simulink model "Three_Phase_Rectifier"  (R2019b)
settings: Solver=ode45  StartTime=0.0  StopTime=2  RelTol=1e-3  EnableMultiTasking=on
libraries: powerlib x21, powerlib_extras x4, eeTransforms x1, simulink x1
settings Model: Creator=Administrator  LastModifiedBy=de
settings DataIOCC: LimitDataPoints=on  SaveFormat=Array  SignalLoggingSaveFormat=ModelDataLogs  ReturnWorkspaceOutputs=off
settings OptimizationCC: ExpressionDepthLimit=2147483647  LifeSpan=inf
settings DebuggingCC: UnderspecifiedInitializationDetection=Classic  MergeDetectMultiDrivingBlocksExec=none  SolverPrmCheckMsg=warning  FcnCallInpInsideContextMsg=warning  StateNameClashWarn=warning  SFUnexpectedBacktrackingDiag=warning  SFNoUnconditionalDefaultTransitionDiag=warning  SFExecutionAtInitializationDiag=none  ArithmeticOperatorsInVariantConditions=warning
settings HardwareCC: ProdBitPerPointer=32  ProdBitPerSizeT=32  ProdBitPerPtrDiffT=32  ProdLargestAtomicFloat=None  ProdIntDivRoundTo=Undefined  ProdEndianess=Unspecified  ProdWordSize=32  ProdHWDeviceType=32-bit Generic
settings ModelReferenceCC: PropagateSignalLabelsOutOfModel=off
settings SFSimCC: SimUseLocalCustomCode=off  CustomCodeUndefinedFunction=UseInterfaceOnly
settings RTWCC: RTWUseLocalCustomCode=off
settings CodeAppCC: StateflowObjectComments=on
settings GRTTargetCC: TargetLangStandard=C89/C90 (ANSI)  GeneratePreprocessorConditionals=Disable all  CombineOutputUpdateFcns=off  GRTInterface=on
settings ConfigComp: CovMetricSettings=dw  CovHtmlReporting=on  CovSaveCumulativeToWorkspaceVar=on  CovSaveSingleToWorkspaceVar=on  CovExternalEMLEnable=off
settings SimscapeCC: SimscapeNormalizeSystem=off

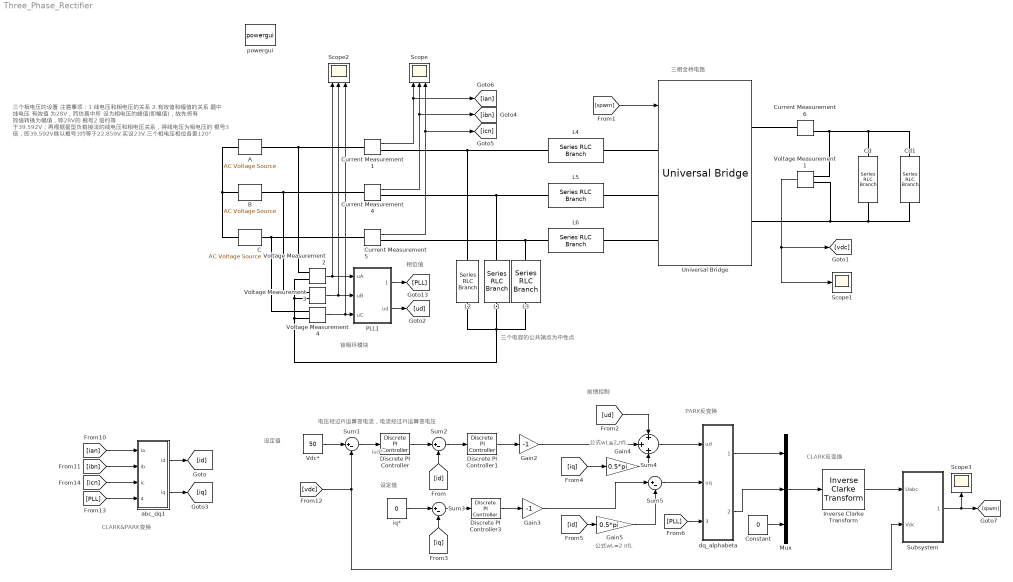
== system Three_Phase_Rectifier ==
  note: 前馈控制
  note: 电压经过PI运算变电流，电流经过PI运算变电压
  note: 公式wL=2 πfL
  note: 相位值
  note: 设定值
  note: CLARK&PARK变换
  note: PARK反变换
  note: 三个电容的公共端点为中性点
  note: isd*
  note: 三个相电压的设置
      | 注意事项：1.线电压和相电压的关系
      | 2.有效值和幅值的关系
      | 题中 线电压 有效值 为28V，而仿真中所
      | 设为相电压的峰值(即幅值)，故先将有
      | 效值转换为幅值，即28V的 根号2 倍约等
      | 于39.592V；再根据星型负载接法的线电压和相电压关系，得线电压为相电压的 根号3 倍，即39.592V除以根号3约等于22.859V,实设23V.三个相电压相位各差120°
  note: 锁相环模块
  note: 三相全桥电路
  note: CLARK反变换
  note: 设定值
  note: 公式wL=2 πfL
  A : powerlib/Electrical Sources/AC Voltage Source  Amplitude=23  Phase=-120  Frequency=50  SampleTime=0  Measurements=None  BusType=swing  Pref=10e3  Qref=0  Qmin=-inf  Qmax=+inf
      settings: SourceProductName=Simscape Electrical
  B : powerlib/Electrical Sources/AC Voltage Source  Amplitude=23  Phase=120  Frequency=50  SampleTime=0  Measurements=None  BusType=swing  Pref=10e3  Qref=0  Qmin=-inf  Qmax=+inf
      settings: SourceProductName=Simscape Electrical
  C : powerlib/Electrical Sources/AC Voltage Source  Amplitude=23  Phase=0  Frequency=50  SampleTime=0  Measurements=None  BusType=swing  Pref=10e3  Qref=0  Qmin=-inf  Qmax=+inf
      settings: SourceProductName=Simscape Electrical
  Cd : powerlib/Elements/Series RLC Branch  LConnTagsString=__new0  RConnTagsString=__new0  BranchType=C  Resistance=100  Inductance=1e-3  SetiL0=off  InitialCurrent=0  Capacitance=1e-3  Setx0=on  InitialVoltage=0  Measurements=None
      settings: SourceProductName=Simscape Electrical
  Cd1 : powerlib/Elements/Series RLC Branch  LConnTagsString=__new0  RConnTagsString=__new0  BranchType=R  Resistance=50  Inductance=1e-3  SetiL0=off  InitialCurrent=0  Capacitance=2e-3  Setx0=on  InitialVoltage=540  Measurements=None
      settings: SourceProductName=Simscape Electrical
  Constant : Constant  Value=0
  Current Measurement{1,4..6} (4 alike) : powerlib/Measurements/Current Measurement  PhasorSimulation=off  OutputType=Complex  PSBequivalent=0
      settings: SourceProductName=Simscape Electrical
  Discrete PI Controller : powerlib_extras/Discrete  Control Blocks/Discrete PI Controller  Kp=0.5  Ki=12  Par_Limits=[30 -30]  Init=0  Ts=1e-6
      settings: SourceProductName=Simscape Electrical
  Discrete PI Controller1 : powerlib_extras/Discrete  Control Blocks/Discrete PI Controller  Kp=1  Ki=0.0001  Par_Limits=[200 -200]  Init=0  Ts=1e-6
      settings: SourceProductName=Simscape Electrical
  Discrete PI Controller3 : powerlib_extras/Discrete  Control Blocks/Discrete PI Controller  Kp=1  Ki=0.0001  Par_Limits=[200 -200]  Init=0  Ts=1e-6
      settings: SourceProductName=Simscape Electrical
  Gain2 : Gain  Gain=-1  SampleTime=1e-4
  Gain3 : Gain  Gain=-1
  Gain4 : Gain  Gain=0.5*pi
  Gain5 : Gain  Gain=0.5*pi
  Inverse Clarke Transform : eeTransforms/Inverse Clarke Transform  PowerInvariant=off
      settings: SourceProductName=Simscape Electrical  SourceProductBaseCode=PS
  L1 : powerlib/Elements/Series RLC Branch  LConnTagsString=__new0  RConnTagsString=__new0  BranchType=RC  Resistance=0.001  Inductance=2e-3  SetiL0=off  InitialCurrent=0  Capacitance=10e-6  Setx0=off  InitialVoltage=0  Measurements=None
      settings: SourceProductName=Simscape Electrical
  L2 : powerlib/Elements/Series RLC Branch  LConnTagsString=__new0  RConnTagsString=__new0  BranchType=RC  Resistance=0.001  Inductance=2e-3  SetiL0=off  InitialCurrent=0  Capacitance=10e-6  Setx0=off  InitialVoltage=0  Measurements=None
      settings: SourceProductName=Simscape Electrical
  L3 : powerlib/Elements/Series RLC Branch  LConnTagsString=__new0  RConnTagsString=__new0  BranchType=RC  Resistance=0.001  Inductance=2e-3  SetiL0=off  InitialCurrent=0  Capacitance=10e-6  Setx0=off  InitialVoltage=0  Measurements=None
      settings: SourceProductName=Simscape Electrical
  L4 : powerlib/Elements/Series RLC Branch  LConnTagsString=__new0  RConnTagsString=__new0  BranchType=L  Resistance=1  Inductance=2e-3  SetiL0=off  InitialCurrent=0  Capacitance=2e-3  Setx0=off  InitialVoltage=0  Measurements=None
      settings: SourceProductName=Simscape Electrical
  L5 : powerlib/Elements/Series RLC Branch  LConnTagsString=__new0  RConnTagsString=__new0  BranchType=L  Resistance=1  Inductance=2e-3  SetiL0=off  InitialCurrent=0  Capacitance=2e-3  Setx0=off  InitialVoltage=0  Measurements=None
      settings: SourceProductName=Simscape Electrical
  L6 : powerlib/Elements/Series RLC Branch  LConnTagsString=__new0  RConnTagsString=__new0  BranchType=L  Resistance=1  Inductance=2e-3  SetiL0=off  InitialCurrent=0  Capacitance=2e-3  Setx0=off  InitialVoltage=0  Measurements=None
      settings: SourceProductName=Simscape Electrical
  Mux : Mux  Inputs=3
  PLL1 : Subsystem
  Scope : Scope  NumInputPorts=3
  Scope1 : Scope
  Scope2 : Scope  NumInputPorts=3
  Scope3 : Scope
  Subsystem : Subsystem
  Sum1 : Sum  Inputs=|+-  SampleTime=1e-4
  Sum2 : Sum  Inputs=|+-
  Sum3 : Sum  Inputs=|+-
  Sum4 : Sum  Inputs=+|+|+  SampleTime=1e-4
  Sum5 : Sum  Inputs=|+-
  Universal Bridge : powerlib/Power Electronics/Universal Bridge  Arms=3  SnubberResistance=1e5  SnubberCapacitance=inf  Device=MOSFET / Diodes  Ron=1e-3  Lon=0  ForwardVoltages="[  0  0  ]"  ForwardVoltage=0  GTOparameters=[ 10e-6 , 20e-6 ]  IGBTparameters=[ 1e-6 , 2e-6 ]  Measurements=None  Measurements_2=None  converterType=Rectifier
      settings: SourceProductName=Simscape Electrical
  Vdc* : Constant  Value=50
  Voltage Measurement{1..4} (4 alike) : powerlib/Measurements/Voltage Measurement  PhasorSimulation=off  OutputType=Complex  PSBequivalent=0
      settings: SourceProductName=Simscape Electrical
  abc_dq1 : Subsystem
  dq_alphabeta : Subsystem
  iq* : Constant  Value=0
  powergui : powerlib/powergui  Priority=1  SimulationMode=Discrete  SampleTime=10e-7  frequency=60  Iterations=50  frequencyindice=0  Pbase=100e6  ErrMax=1e-4  UnitsV=kV  UnitsW=MW  buscounter=0  FunctionMessages=off  echomessages=off  EnableUseOfTLC=off  CurrentSourceSwitches=off  DisableSnubberDevices=off  DisableRonSwitches=off  DisableVfSwitches=off  DisplayEquations=off  AutomaticDiscreteSolvers=off  SolverType=Tustin  Interpol=off  ExternalGateDelay=off  methode=off  Ts=0  x0status=blocks  SPID=off  SwTol=0  HookPort=off  NonlinearTolerance=1e-4  nMaxIteration=100  ContinueOnMaxIteration=off  RestoreLinks=warning  ResistiveCurrentMeasurement=off  Frange=[0:2:500]  Ylog=off  Xlog=on  ShowGrid=off  save=off  variable=ZData  structure=0  ZoomFFT=off  StartTime=0.0  cycles=1  DisplayStyle=1  fundamental=60  FreqAxis=off  MaxFrequency=1000  frequencyindicesteady=1  RmsSteady=1  display=off
      settings: SourceProductName=Simscape Electrical
  wires:
  Voltage Measurement3/1 -> Scope2/2, PLL1/2(uB)
  Voltage Measurement4/1 -> Scope2/3, PLL1/3(uC)
  Voltage Measurement2/1 -> Scope2/1, PLL1/1(uA)
  PLL1/1(theta_pll) -> [PLL]
  PLL1/2(ud) -> [ud]
  [ian] -> abc_dq1/1(ia)
  [icn] -> abc_dq1/3(ic)
  [ibn] -> abc_dq1/2(ib)
  [spwm] -> Universal Bridge/1
  [ud] -> Sum4/1
  Vdc*/1 -> Sum1/1
  [PLL] -> abc_dq1/4(theta)
  Sum1/1 -> Discrete PI Controller/1
  Discrete PI Controller/1 -> Sum2/1
  iq*/1 -> Sum3/1
  Sum3/1 -> Discrete PI Controller3/1
  Sum2/1 -> Discrete PI Controller1/1
  Discrete PI Controller1/1 -> Gain2/1
  Discrete PI Controller3/1 -> Gain3/1
  Gain2/1 -> Sum4/2
  Gain3/1 -> Sum5/1
  Gain4/1 -> Sum4/3
  Gain5/1 -> Sum5/2
  dq_alphabeta/1(ualpha) -> Mux/1
  dq_alphabeta/2(ubeta) -> Mux/2
  Sum4/1 -> dq_alphabeta/1(ud)
  Sum5/1 -> dq_alphabeta/2(uq)
  abc_dq1/2(iq) -> [iq]
  [vdc] -> Sum1/2, Subsystem/2("Vdc ")
  Current Measurement4/1 -> Scope/2, [ibn]
  Current Measurement5/1 -> Scope/3, [icn]
  Mux/1 -> Inverse Clarke Transform/1
  Inverse Clarke Transform/1 -> Subsystem/1(Uabc)
  Subsystem/1(SPWM) -> [spwm], Scope3/1
  Constant/1 -> Mux/3
  abc_dq1/1(id) -> [id]
  Current Measurement1/1 -> Scope/1, [ian]
  Voltage Measurement1/1 -> Scope1/1, [vdc]
  [id] -> Sum2/2
  [iq] -> Sum3/2
  [iq] -> Gain4/1
  [id] -> Gain5/1
  [PLL] -> dq_alphabeta/3(theta)
  connections:
  C/RConn1 -- Current Measurement5/LConn1 -- Voltage Measurement4/LConn1
  Voltage Measurement3/LConn1 -- Current Measurement4/LConn1 -- B/RConn1
  Universal Bridge/LConn3 -- L6/RConn1
  Universal Bridge/LConn2 -- L5/RConn1
  Cd1/LConn1 -- Voltage Measurement1/LConn1 -- Current Measurement6/RConn1 -- Cd/LConn1
  Universal Bridge/RConn2 -- Voltage Measurement1/LConn2 -- Cd1/RConn1 -- Cd/RConn1
  C/LConn1 -- A/LConn1 -- B/LConn1
  Universal Bridge/LConn1 -- L4/RConn1
  Current Measurement1/RConn1 -- L4/LConn1 -- L2/LConn1
  Current Measurement4/RConn1 -- L5/LConn1 -- L1/LConn1
  Current Measurement5/RConn1 -- L6/LConn1 -- L3/LConn1
  Current Measurement6/LConn1 -- Universal Bridge/RConn1
  L1/RConn1 -- L3/RConn1 -- Voltage Measurement2/LConn2 -- Voltage Measurement3/LConn2 -- Voltage Measurement4/LConn2 -- L2/RConn1
  A/RConn1 -- Current Measurement1/LConn1 -- Voltage Measurement2/LConn1

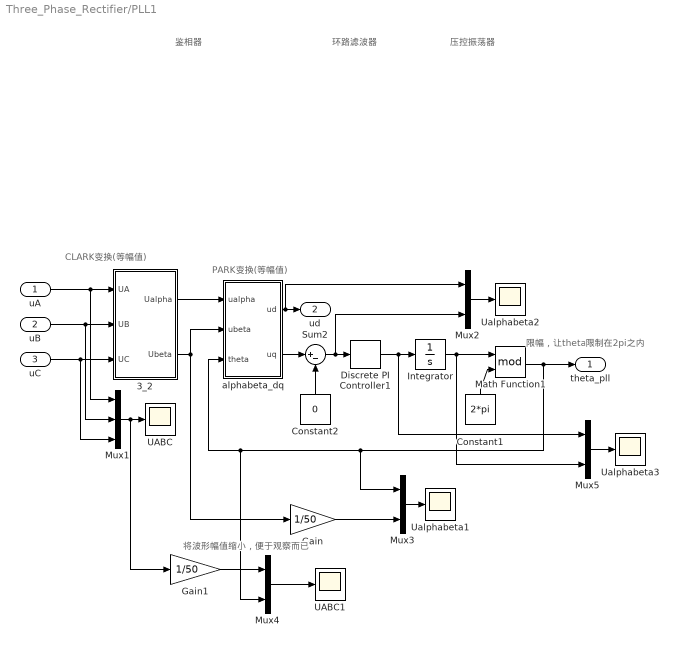
== system Three_Phase_Rectifier/PLL1 ==
  note: 压控振荡器
  note: 环路滤波器
  note: 鉴相器
  note: 限幅，让theta限制在2pi之内
  note: 将波形幅值缩小，便于观察而已
  note: CLARK变换(等幅值)
  note: PARK变换(等幅值)
  uA : Inport
  uB : Inport  Port=2
  uC : Inport  Port=3
  3_2 : Subsystem
  Constant1 : Constant  Value=2*pi
  Constant2 : Constant  Value=0
  Discrete PI Controller1 : powerlib_extras/Discrete  Control Blocks/Discrete PI Controller  Kp=20  Ki=120  Par_Limits=[1e6 -1e6]  Init=0  Ts=1e-6
      settings: SourceProductName=Simscape Electrical
  Gain : Gain  Gain=1/50
  Gain1 : Gain  Gain=1/50
  Integrator : Integrator
  Math Function1 : Math  Operator=mod  SaturateOnIntegerOverflow=on
  Mux1 : Mux  Inputs=3
  Mux{2..5} (4 alike) : Mux  Inputs=2
  Sum2 : Sum  Inputs=|+-
  UABC : Scope
  UABC1 : Scope
  Ualphabeta1 : Scope
  Ualphabeta2 : Scope
  Ualphabeta3 : Scope
  alphabeta_dq : Subsystem
  theta_pll : Outport
  ud : Outport  Port=2
  wires:
  Gain1/1 -> Mux4/1
  Mux4/1 -> UABC1/1
  Gain/1 -> Mux3/2
  Mux3/1 -> Ualphabeta1/1
  Math Function1/1 -> theta_pll/1, Mux3/1, Mux4/2, alphabeta_dq/3(theta)
  Constant1/1 -> Math Function1/2
  Discrete PI Controller1/1 -> Mux5/1, Integrator/1
  alphabeta_dq/2(uq) -> Sum2/1
  3_2/2(Ubeta) -> Gain/1, alphabeta_dq/2(ubeta)
  3_2/1(Ualpha) -> alphabeta_dq/1(ualpha)
  uC/1 -> 3_2/3(UC), Mux1/3
  uB/1 -> 3_2/2(UB), Mux1/2
  uA/1 -> 3_2/1(UA), Mux1/1
  Mux1/1 -> Gain1/1, UABC/1
  Sum2/1 -> Mux2/2, Discrete PI Controller1/1
  Constant2/1 -> Sum2/2
  alphabeta_dq/1(ud) -> Mux2/1, ud/1
  Mux2/1 -> Ualphabeta2/1
  Mux5/1 -> Ualphabeta3/1
  Integrator/1 -> Math Function1/1, Mux5/2

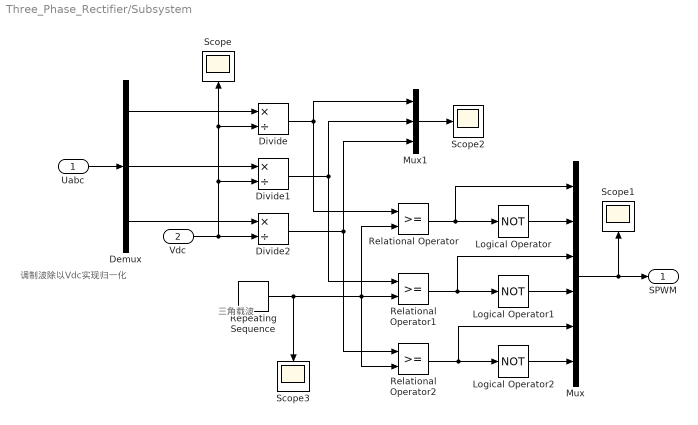
== system Three_Phase_Rectifier/Subsystem ==
  note: 调制波除以Vdc实现归一化
  note: 三角载波
  Uabc : Inport
  "Vdc " : Inport  Port=2
  Demux : Demux  Outputs=3
  Divide : Product  Inputs=*/
  Divide1 : Product  Inputs=*/
  Divide2 : Product  Inputs=*/
  Logical Operator : Logic  Operator=NOT  AllPortsSameDT=off  OutDataTypeStr=boolean
  Logical Operator1 : Logic  Operator=NOT  AllPortsSameDT=off  OutDataTypeStr=boolean
  Logical Operator2 : Logic  Operator=NOT  AllPortsSameDT=off  OutDataTypeStr=boolean
  Mux : Mux  Inputs=6
  Mux1 : Mux  Inputs=3
  Relational Operator : RelationalOperator  OutDataTypeStr=boolean  RndMeth=Simplest
  Relational Operator1 : RelationalOperator  OutDataTypeStr=boolean  RndMeth=Simplest
  Relational Operator2 : RelationalOperator  OutDataTypeStr=boolean  RndMeth=Simplest
  Repeating Sequence : simulink/Sources/Repeating Sequence  rep_seq_t=[0 2.5e-5 5e-5]  rep_seq_y=[-1 1 -1]
  Scope{,1..3} (4 alike) : Scope
  SPWM : Outport
  wires:
  Uabc/1 -> Demux/1
  Repeating Sequence/1 -> Scope3/1, Relational Operator2/2, Relational Operator/2, Relational Operator1/2
  Demux/1 -> Divide/1
  Divide/1 -> Relational Operator/1, Mux1/1
  Demux/2 -> Divide1/1
  Demux/3 -> Divide2/1
  "Vdc "/1 -> Divide2/2, Divide/2, Scope/1, Divide1/2
  Divide1/1 -> Relational Operator1/1, Mux1/2
  Divide2/1 -> Mux1/3, Relational Operator2/1
  Mux/1 -> Scope1/1, SPWM/1
  Relational Operator/1 -> Mux/1, Logical Operator/1
  Logical Operator/1 -> Mux/2
  Relational Operator1/1 -> Mux/3, Logical Operator1/1
  Logical Operator1/1 -> Mux/4
  Relational Operator2/1 -> Mux/5, Logical Operator2/1
  Logical Operator2/1 -> Mux/6
  Mux1/1 -> Scope2/1

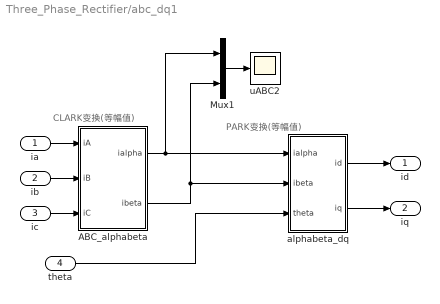
== system Three_Phase_Rectifier/abc_dq1 ==
  note: CLARK变换(等幅值)
  note: PARK变换(等幅值)
  ia : Inport
  ib : Inport  Port=2
  ic : Inport  Port=3
  theta : Inport  Port=4
  ABC_alphabeta : Subsystem
  Mux1 : Mux  Inputs=2
  alphabeta_dq : Subsystem
  uABC2 : Scope
  id : Outport
  iq : Outport  Port=2
  wires:
  Mux1/1 -> uABC2/1
  theta/1 -> alphabeta_dq/3(theta)
  alphabeta_dq/1(id) -> id/1
  alphabeta_dq/2(iq) -> iq/1
  ABC_alphabeta/2(ibeta) -> Mux1/2, alphabeta_dq/2(ibeta)
  ABC_alphabeta/1(ialpha) -> Mux1/1, alphabeta_dq/1(ialpha)
  ib/1 -> ABC_alphabeta/2(iB)
  ia/1 -> ABC_alphabeta/1(iA)
  ic/1 -> ABC_alphabeta/3(iC)

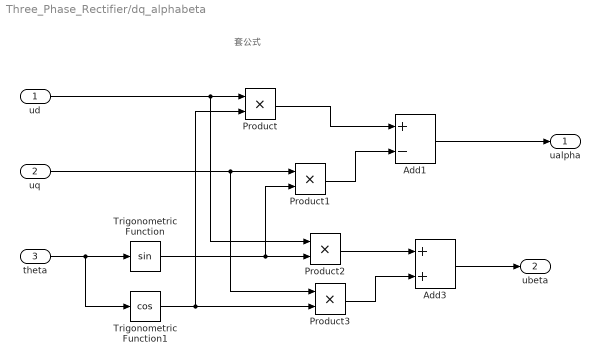
== system Three_Phase_Rectifier/dq_alphabeta ==
  note: 套公式
  ud : Inport
  uq : Inport  Port=2
  theta : Inport  Port=3
  Add1 : Sum  Inputs=+-
  Add3 : Sum
  Product{,1..3} (4 alike) : Product  RndMeth=Zero
  Trigonometric Function : Trigonometry
  Trigonometric Function1 : Trigonometry  Operator=cos
  ualpha : Outport
  ubeta : Outport  Port=2
  wires:
  theta/1 -> Trigonometric Function/1, Trigonometric Function1/1
  ud/1 -> Product/1, Product2/1
  Product/1 -> Add1/1
  Product1/1 -> Add1/2
  Add1/1 -> ualpha/1
  Product2/1 -> Add3/1
  Product3/1 -> Add3/2
  Add3/1 -> ubeta/1
  Trigonometric Function1/1 -> Product/2, Product3/2
  uq/1 -> Product1/1, Product3/1
  Trigonometric Function/1 -> Product1/2, Product2/2

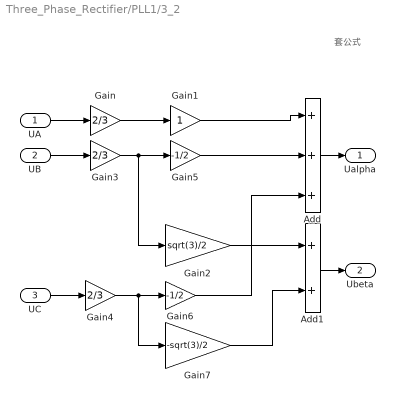
== system Three_Phase_Rectifier/PLL1/3_2 ==
  note: 套公式
  UA : Inport
  UB : Inport  Port=2
  UC : Inport  Port=3
  Add : Sum  Inputs=+++
  Add1 : Sum
  Gain : Gain  Gain=2/3
  Gain1 : Gain
  Gain2 : Gain  Gain=sqrt(3)/2
  Gain3 : Gain  Gain=2/3
  Gain4 : Gain  Gain=2/3
  Gain5 : Gain  Gain=-1/2
  Gain6 : Gain  Gain=-1/2
  Gain7 : Gain  Gain=-sqrt(3)/2
  Ualpha : Outport
  Ubeta : Outport  Port=2
  wires:
  UA/1 -> Gain/1
  UB/1 -> Gain3/1
  UC/1 -> Gain4/1
  Gain4/1 -> Gain7/1, Gain6/1
  Gain3/1 -> Gain2/1, Gain5/1
  Gain/1 -> Gain1/1
  Gain1/1 -> Add/1
  Gain5/1 -> Add/2
  Gain6/1 -> Add/3
  Add/1 -> Ualpha/1
  Add1/1 -> Ubeta/1
  Gain2/1 -> Add1/1
  Gain7/1 -> Add1/2

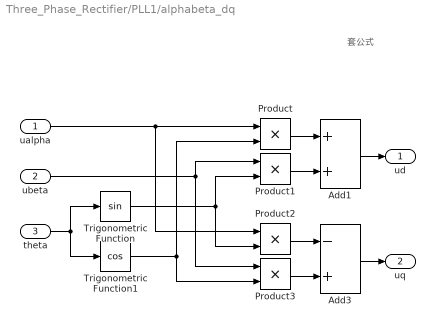
== system Three_Phase_Rectifier/PLL1/alphabeta_dq ==
  note: 套公式
  ualpha : Inport
  ubeta : Inport  Port=2
  theta : Inport  Port=3
  Add1 : Sum  SampleTime=1e-4
  Add3 : Sum  Inputs=-+  SampleTime=1e-4
  Product{,1..3} (4 alike) : Product  SampleTime=1e-4  RndMeth=Zero
  Trigonometric Function : Trigonometry  SampleTime=1e-4
  Trigonometric Function1 : Trigonometry  Operator=cos  SampleTime=1e-4
  ud : Outport
  uq : Outport  Port=2
  wires:
  theta/1 -> Trigonometric Function1/1, Trigonometric Function/1
  ualpha/1 -> Product/1, Product2/1
  Trigonometric Function1/1 -> Product3/2, Product/2
  ubeta/1 -> Product1/1, Product3/1
  Trigonometric Function/1 -> Product2/2, Product1/2
  Product/1 -> Add1/1
  Product1/1 -> Add1/2
  Add1/1 -> ud/1
  Product2/1 -> Add3/1
  Product3/1 -> Add3/2
  Add3/1 -> uq/1

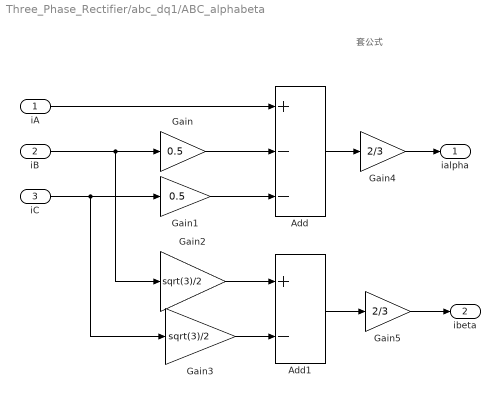
== system Three_Phase_Rectifier/abc_dq1/ABC_alphabeta ==
  note: 套公式
  iA : Inport
  iB : Inport  Port=2
  iC : Inport  Port=3
  Add : Sum  Inputs=+--
  Add1 : Sum  Inputs=+-
  Gain : Gain  Gain=0.5
  Gain1 : Gain  Gain=0.5
  Gain2 : Gain  Gain=sqrt(3)/2
  Gain3 : Gain  Gain=sqrt(3)/2
  Gain4 : Gain  Gain=2/3
  Gain5 : Gain  Gain=2/3
  ialpha : Outport
  ibeta : Outport  Port=2
  wires:
  iB/1 -> Gain/1, Gain2/1
  iC/1 -> Gain3/1, Gain1/1
  Gain/1 -> Add/2
  Gain1/1 -> Add/3
  iA/1 -> Add/1
  Add/1 -> Gain4/1
  Gain2/1 -> Add1/1
  Gain3/1 -> Add1/2
  Add1/1 -> Gain5/1
  Gain4/1 -> ialpha/1
  Gain5/1 -> ibeta/1

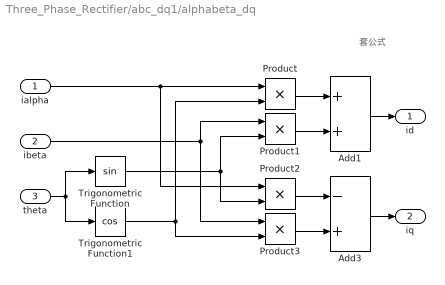
== system Three_Phase_Rectifier/abc_dq1/alphabeta_dq ==
  note: 套公式
  ialpha : Inport
  ibeta : Inport  Port=2
  theta : Inport  Port=3
  Add1 : Sum
  Add3 : Sum  Inputs=-+
  Product{,1..3} (4 alike) : Product  RndMeth=Zero
  Trigonometric Function : Trigonometry
  Trigonometric Function1 : Trigonometry  Operator=cos
  id : Outport
  iq : Outport  Port=2
  wires:
  Add3/1 -> iq/1
  Product3/1 -> Add3/2
  Product2/1 -> Add3/1
  Add1/1 -> id/1
  Product1/1 -> Add1/2
  Product/1 -> Add1/1
  Trigonometric Function/1 -> Product2/2, Product1/2
  ibeta/1 -> Product3/1, Product1/1
  Trigonometric Function1/1 -> Product3/2, Product/2
  ialpha/1 -> Product2/1, Product/1
  theta/1 -> Trigonometric Function1/1, Trigonometric Function/1
